simulink model "lab3s2022a"  (R2022a)
settings: Solver=VariableStepAuto  StartTime=0.0  StopTime=250  RelTol=1e-3
values from neighbouring files (symbols this model uses):
  A = [-Ra/La -psi/La 0 0; psi/JM -b/JM b/JM -1/JM; 0 b/JL -b/JL 1/JL; 0 k -k 0]    [lab3m.m]
  b = 0.06    [lab3m.m]
  B = [1/La; 0; 0; 0;]    [lab3m.m]
  C = [0 1 0 0]    [lab3m.m]
  D = 0    [lab3m.m]
  JL = 0.00450213442287325    (= 0.00450213442287)    [lab3m.m]
  JM = 0.00150071147429108    (= 0.00150071147429)    [lab3m.m]
  k = 1700    [lab3m.m]
  La = 0.00035    [lab3m.m]
  psi = 0.229183118052329    (= 0.229183118052)    [lab3m.m]
  Ra = 0.35    [lab3m.m]
  U = U_rated    (= 24)    [lab3m.m]
libraries: fl_lib x9, nesl_utility x5, simulink x1, ee_lib x1
settings Model: Creator=86156  LastModifiedBy=86156
settings ModelReferenceCC: EnableRefExpFcnMdlSchedulingChecks=off
settings RTWCC: Description=Generic Real-Time Target

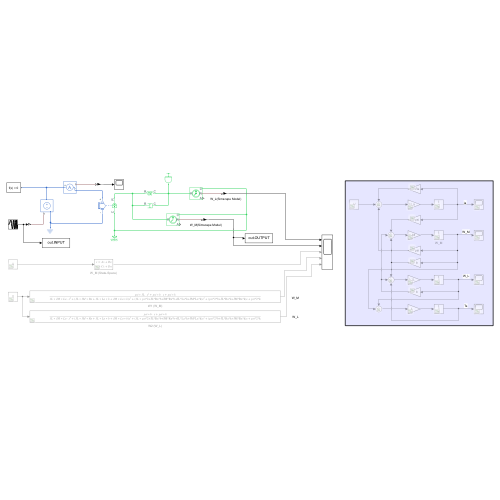
[thumbnail: Simulink's stored preview of the top-level diagram]
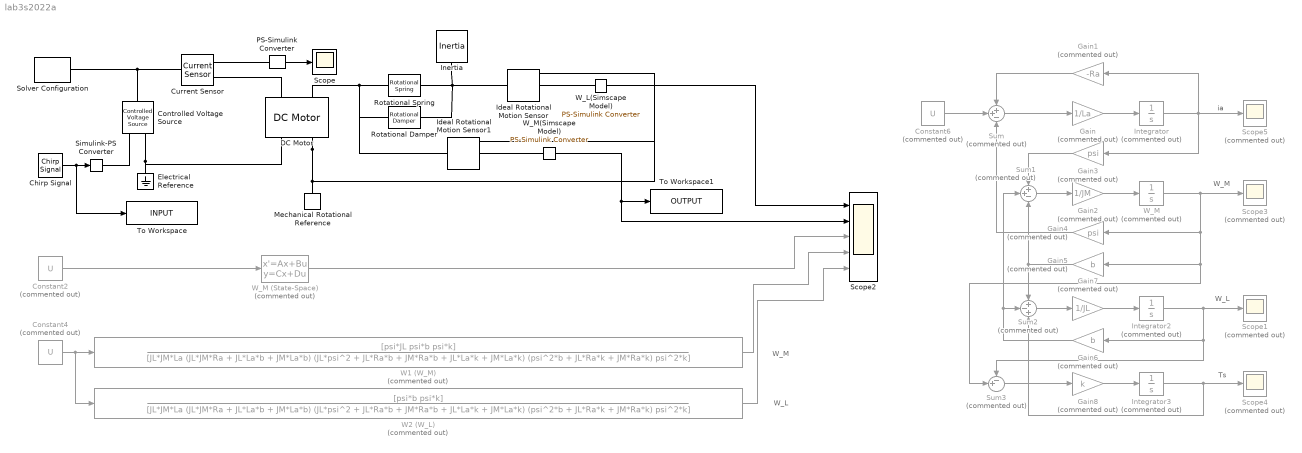
== system lab3s2022a ==
  note: Ts
  note: W_L
  note: W_M
  note: ia
  note: W_M
  note: W_L
  Chirp Signal : simulink/Sources/Chirp Signal  f1=0.1  T=250  f2=500
  Constant2 : Constant  Commented=on  Value=U
  Constant4 : Constant  Commented=on  Value=U
  Constant6 : Constant  Commented=on  Value=U
  Controlled Voltage Source : fl_lib/Electrical/Electrical Sources/Controlled Voltage Source
  Current Sensor : fl_lib/Electrical/Electrical Sensors/Current Sensor
  DC Motor : ee_lib/Electromechanical/Brushed Motors/DC Motor  field_option=ee.enum.field_option.pm  Rf=100 Ohm  Lf=1 H  Laf=0.15 H  If0=0 A  parameterization=ee.enum.dcparam_option.circuit_param  Ra=Ra Ohm  La=La H  emf_or_torque=ee.enum.emf_or_torque.kv  Kv=psi V/(rad/s)  Ki=6.876e-4 N*m/A  T_stall=0.24e-3 N*m  w_max=19100 rpm  w_rated=15000 rpm  P_rated=0.08 W  V_rated=1.5 V  lam_param=ee.enum.lam_param.damping  i_noload=0 A  V_i_noload=1.5 V  J=JM kg*m^2  lam=0 N*m/(rad/s)  speed0=0 rpm  enable_fault_armature=simscape.enum.onoff.off  rev_faulted=1 / 3  G_faulted_armature=1e-5 S  fault_trigger_armature=ee.enum.faults.faultTrigger.temporal  t_fault_armature=1 s  max_permissible_current_armature=inf A  t_fail_on_current_armature=1 s  enable_fault_field=simscape.enum.onoff.off  G_faulted_field=1e-5 S  fault_trigger_field=ee.enum.faults.faultTrigger.temporal  t_fault_field=1 s  max_permissible_current_field=inf A  t_fail_on_current_field=1 s  fault_action=simscape.enum.assert.action.none  alpha=3.93e-3 1/K  Tmeas=25 degC  thermal_mass=100 J/K  initial_temperature=25 degC
  Electrical Reference : fl_lib/Electrical/Electrical Elements/Electrical Reference
  Gain : Gain  Commented=on  Gain=1/La
  Gain1 : Gain  Commented=on  Gain=-Ra
  Gain2 : Gain  Commented=on  Gain=1/JM
  Gain3 : Gain  Commented=on  Gain=psi
  Gain4 : Gain  Commented=on  Gain=psi
  Gain5 : Gain  Commented=on  Gain=b
  Gain6 : Gain  Commented=on  Gain=b
  Gain7 : Gain  Commented=on  Gain=1/JL
  Gain8 : Gain  Commented=on  Gain=k
  Ideal Rotational Motion Sensor : fl_lib/Mechanical/Mechanical Sensors/Ideal Rotational Motion Sensor  reference=foundation.enum.MeasurementReference.difference  acceleration_port=false  velocity_port=true  position_port=true  wrap_angle=false  offset=0 rad
  Ideal Rotational Motion Sensor1 : fl_lib/Mechanical/Mechanical Sensors/Ideal Rotational Motion Sensor  reference=foundation.enum.MeasurementReference.difference  acceleration_port=false  velocity_port=true  position_port=true  wrap_angle=false  offset=0 rad
  Inertia : fl_lib/Mechanical/Rotational Elements/Inertia  inertia=JL kg*m^2  num_ports=foundation.enum.numPorts2.one  w_specify=off  w_priority=High  w=0 rad/s  w_nominal_specify=off  w_nominal_unit=rad/s  w_nominal_value=1  t_specify=off  t_priority=None  t=0 N*m  t_nominal_specify=off  t_nominal_unit=N*m  t_nominal_value=1
  Integrator : Integrator  Commented=on
  Integrator2 : Integrator  Commented=on
  Integrator3 : Integrator  Commented=on
  Mechanical Rotational Reference : fl_lib/Mechanical/Rotational Elements/Mechanical Rotational Reference
  PS-Simulink Converter : nesl_utility/PS-Simulink Converter  PhysicalDomain=network_engine_domain  SubClassName=ps_output  LeftPortType=input  RightPortType=output  PseudoPeriodic=off  Frequencies=[]  VectorFormat=inherit  Unit=inherit  AffineConversion=off
  Rotational Damper : fl_lib/Mechanical/Rotational Elements/Rotational Damper  D=b N*m*s/rad  w_specify=off  w_priority=None  w=0 rad/s  w_nominal_specify=off  w_nominal_unit=rad/s  w_nominal_value=1  t_specify=off  t_priority=None  t=0 N*m  t_nominal_specify=off  t_nominal_unit=N*m  t_nominal_value=1
  Rotational Spring : fl_lib/Mechanical/Rotational Elements/Rotational Spring  spr_rate=k N*m/rad  w_specify=off  w_priority=None  w=0 rad/s  w_nominal_specify=off  w_nominal_unit=rad/s  w_nominal_value=1  t_specify=off  t_priority=None  t=0 N*m  t_nominal_specify=off  t_nominal_unit=N*m  t_nominal_value=1  phi_specify=off  phi_priority=High  phi=0 rad  phi_nominal_specify=off  phi_nominal_unit=rad  phi_nominal_value=1
  Scope : Scope
  Scope{1,3..5} (4 alike) : Scope  Commented=on
  Scope2 : Scope  NumInputPorts=5
  Simulink-PS Converter : nesl_utility/Simulink-PS Converter  PhysicalDomain=network_engine_domain  SubClassName=ps_input  LeftPortType=input  RightPortType=output  PseudoPeriodic=off  Frequencies=[]  NoiseDistribution=none  NoiseParameters=[]  Unit=1  AffineConversion=off  FilteringAndDerivatives=provide  SimscapeFilterOrder=1  InputFilterTimeConstant=0.001  UdotUserProvided=0
  Solver Configuration : nesl_utility/Solver Configuration  PhysicalDomain=network_engine_domain  SubClassName=solver  LeftPortType=input  RightPortType=generic  Tones=[]  Harmonics=[]  SimulateNoise=off  Profile=off  UseLocalSampling=off  EnableSwitchedLinearOptims=on  FrequencyDomain=off  UseCCode=off  RelTol=0.001  AbsTol=0.001  MinStep=1e-09  ToWorkspace=off  RevertToSquareIcSolve=off  NumHomotopyIterations=100  PhasorMode=off  PhasorModeNumHarmonics=1  ConsistencySolver=NEWTON_XTOL_AFTER_FTOL  IndexReductionMethod=DerivativeReplacement  DoDC=off  ResidualTolerance=1e-09  ConsistencyTolSource=GLOBAL  ConsistencyAbsTol=0.001  ConsistencyRelTol=0.001  ConsistencyTolFactor=0.001  UseLocalSolver=off  LocalSolverChoice=NE_BACKWARD_EULER_ADVANCER  ResolveIndetEquations=on  FunctionEvalNumThread=1  LocalSolverSampleTime=0.001  DoFixedCost=off  MaxNonlinIter=3  MaxModeIter=2  ComputeImpulses=off  ImpulseIterations=2  LinearAlgebra=auto  LinearAlgebraNumThread=0  EquationFormulation=NE_TIME_EF  DelaysMemoryBudget=1024  AutomaticFiltering=on  FilteringTimeConstant=0.001  PartitionStorageMethod=AS_NEEDED  PartitionMemoryBudget=1024  PartitionMethod=ROBUST
  Sum : Sum  Commented=on  Inputs=++-
  Sum1 : Sum  Commented=on  Inputs=++-
  Sum2 : Sum  Commented=on  Inputs=+-+
  Sum3 : Sum  Commented=on  Inputs=-+|
  To Workspace : ToWorkspace  VariableName=INPUT  SampleTime=.001
  To Workspace1 : ToWorkspace  VariableName=OUTPUT  SampleTime=.001
  W1 (W_M) : TransferFcn  Commented=on  Numerator=[psi*JL psi*b psi*k]  Denominator=[JL*JM*La (JL*JM*Ra + JL*La*b + JM*La*b) (JL*psi^2 + JL*Ra*b + JM*Ra*b + JL*La*k + JM*La*k) (psi^2*b + JL*Ra*k + JM*Ra*k) psi^2*k]
  W2 (W_L) : TransferFcn  Commented=on  Numerator=[psi*b psi*k]  Denominator=[JL*JM*La (JL*JM*Ra + JL*La*b + JM*La*b) (JL*psi^2 + JL*Ra*b + JM*Ra*b + JL*La*k + JM*La*k) (psi^2*b + JL*Ra*k + JM*Ra*k) psi^2*k]
  W_L(Simscape Model) : nesl_utility/PS-Simulink Converter  PhysicalDomain=network_engine_domain  SubClassName=ps_output  LeftPortType=input  RightPortType=output  PseudoPeriodic=off  Frequencies=[]  VectorFormat=inherit  Unit=inherit  AffineConversion=off
  W_M : Integrator  Commented=on
  W_M (State-Space) : StateSpace  Commented=on  A=A  B=B  C=C  D=D  InitialCondition=0
  W_M(Simscape Model) : nesl_utility/PS-Simulink Converter  PhysicalDomain=network_engine_domain  SubClassName=ps_output  LeftPortType=input  RightPortType=output  PseudoPeriodic=off  Frequencies=[]  VectorFormat=inherit  Unit=inherit  AffineConversion=off
  wires:
  W_M (State-Space)/1 -> Scope2/3
  W2 (W_L)/1 -> Scope2/5
  Sum/1 -> Gain/1
  Constant2/1 -> W_M (State-Space)/1
  W1 (W_M)/1 -> Scope2/4
  Chirp Signal/1 -> To Workspace/1, Simulink-PS Converter/1
  Constant6/1 -> Sum/2
  Constant4/1 -> W2 (W_L)/1, W1 (W_M)/1
  Gain4/1 -> Sum/3
  Gain2/1 -> W_M/1
  Gain1/1 -> Sum/1
  Gain/1 -> Integrator/1
  PS-Simulink Converter/1 -> Scope/1
  Gain3/1 -> Sum1/1
  Sum1/1 -> Gain2/1
  Integrator/1 -> Gain3/1, Scope5/1, Gain1/1
  W_M/1 -> Scope3/1, Sum3/2, Gain5/1, Gain4/1
  W_L(Simscape Model)/1 -> Scope2/1
  W_M(Simscape Model)/1 -> Scope2/2, To Workspace1/1
  Gain5/1 -> Sum2/1, Sum1/3
  Integrator2/1 -> Scope1/1, Gain6/1, Sum3/1
  Sum2/1 -> Gain7/1
  Gain7/1 -> Integrator2/1
  Gain6/1 -> Sum2/2, Sum1/2
  Integrator3/1 -> Scope4/1, Sum2/3
  Sum3/1 -> Gain8/1
  Gain8/1 -> Integrator3/1
  connections:
  Rotational Spring/RConn1 -- Rotational Damper/RConn1 -- Inertia/LConn1 -- Ideal Rotational Motion Sensor/LConn1
  Electrical Reference/LConn1 -- DC Motor/RConn1 -- Controlled Voltage Source/RConn2
  Current Sensor/LConn1 -- Solver Configuration/RConn1 -- Controlled Voltage Source/LConn1
  DC Motor/RConn2 -- Ideal Rotational Motion Sensor1/RConn1 -- Ideal Rotational Motion Sensor/RConn1 -- Mechanical Rotational Reference/LConn1
  Current Sensor/RConn1 -- PS-Simulink Converter/LConn1
  W_L(Simscape Model)/LConn1 -- Ideal Rotational Motion Sensor/RConn2
  Simulink-PS Converter/RConn1 -- Controlled Voltage Source/RConn1
  DC Motor/LConn1 -- Current Sensor/RConn2
  DC Motor/LConn2 -- Ideal Rotational Motion Sensor1/LConn1 -- Rotational Damper/LConn1 -- Rotational Spring/LConn1
  Ideal Rotational Motion Sensor1/RConn2 -- W_M(Simscape Model)/LConn1
